simulink model "R_load"  (R2024a)
settings: Solver=VariableStepAuto  StartTime=0.0  StopTime=1800  RelTol=1e-3
libraries: simulink x1
settings Model: Creator=emanuele  LastModifiedBy=emanuele

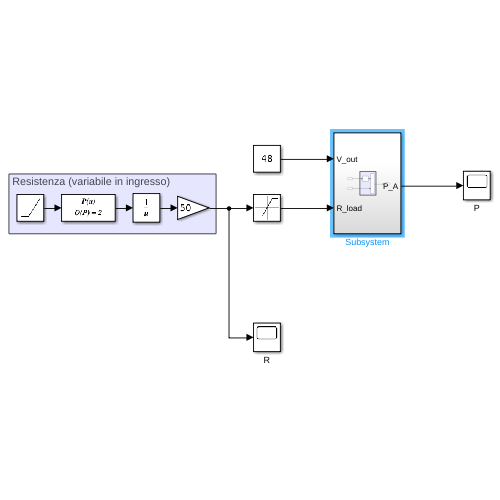
[thumbnail: Simulink's stored preview of the top-level diagram]
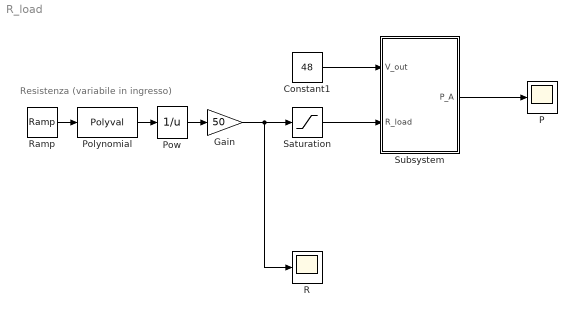
== system R_load ==
  note: Resistenza (variabile in ingresso)
  Constant1 : Constant  Value=48
  Gain : Gain  Gain=50
  P : Scope
  Polynomial : Polyval  Coefs=[10e-4 0 0]
  Pow : Math  Operator=reciprocal  SignedPower=on  RndMeth=Zero
  R : Scope
  Ramp : simulink/Sources/Ramp  slope=0.12  start=10  InitialOutput=0
  Saturation : Saturate  UpperLimit=230  LowerLimit=1.5
  Subsystem : Subsystem
  wires:
  Ramp/1 -> Polynomial/1
  Polynomial/1 -> Pow/1
  Pow/1 -> Gain/1
  Gain/1 -> Saturation/1, R/1
  Constant1/1 -> Subsystem/1(V_out)
  Saturation/1 -> Subsystem/2(R_load)
  Subsystem/1(P_A) -> P/1

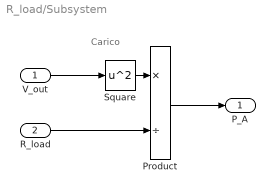
== system R_load/Subsystem ==
  note: Carico
  V_out : Inport  Unit=V
  R_load : Inport  Port=2  Unit=Ω
  Product : Product  Inputs=*/
  Square : Math  Operator=square
  P_A : Outport  Unit=W
  wires:
  Square/1 -> Product/1
  R_load/1 -> Product/2
  Product/1 -> P_A/1
  V_out/1 -> Square/1
